simulink model "ekf_simulation"  (R2023a)
settings: Solver=VariableStepAuto  StartTime=0.0  StopTime=3000  RelTol=1e-3  EnableMultiTasking=on
libraries: aausat3_lib x6, simulink_extras x1
settings Model: Creator=brian  LastModifiedBy=jacobel-omar
settings SolverCC: AlgebraicLoopSolver=TrustRegion
settings DataIOCC: SaveFormat=Array  ReturnWorkspaceOutputs=off
settings OptimizationCC: LifeSpan=inf
settings DebuggingCC: SolverPrmCheckMsg=warning  UnconnectedInputMsg=warning  UnconnectedOutputMsg=warning  UnconnectedLineMsg=warning  AllowSymbolicDim=off  SFUnexpectedBacktrackingDiag=warning  SFNoUnconditionalDefaultTransitionDiag=warning  SFExecutionAtInitializationDiag=none  ArithmeticOperatorsInVariantConditions=warning
settings ModelReferenceCC: EnableRefExpFcnMdlSchedulingChecks=on  PropagateSignalLabelsOutOfModel=off
settings SFSimCC: SimUseLocalCustomCode=off  CustomCodeUndefinedFunction=UseInterfaceOnly
settings RTWCC: RTWUseLocalCustomCode=off
settings CodeAppCC: StateflowObjectComments=on
settings GRTTargetCC: TargetLangStandard=C89/C90 (ANSI)
settings ConfigComp: CovMetricSettings=dw  CovSaveCumulativeToWorkspaceVar=on  CovSaveSingleToWorkspaceVar=on  CovExternalEMLEnable=off  CovSFcnEnable=off

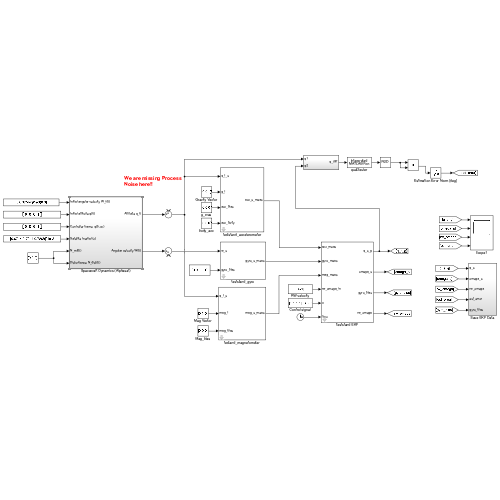
[thumbnail: Simulink's stored preview of the top-level diagram]
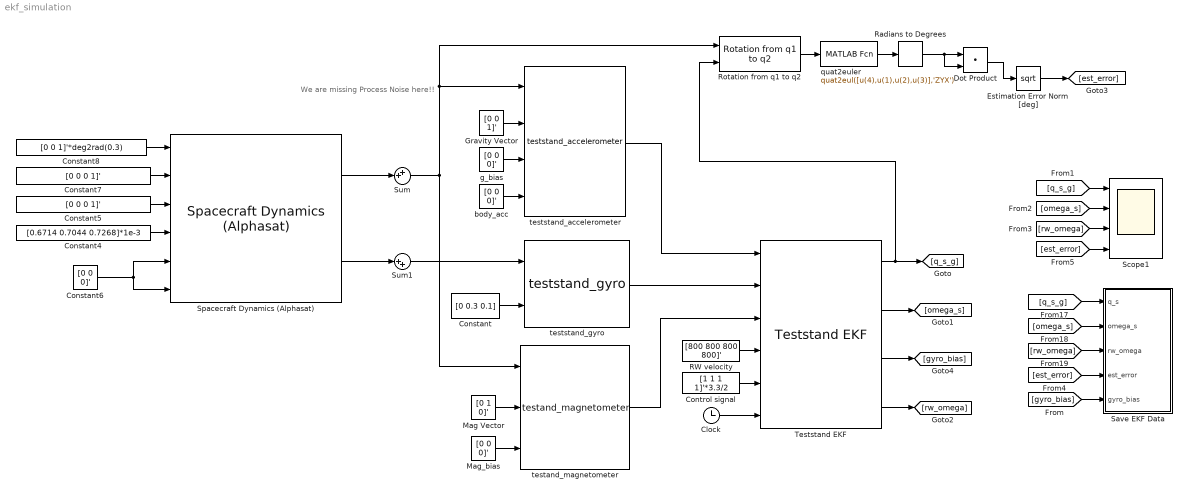
== system ekf_simulation ==
  note: We are missing Process
      | Noise here!!
  Clock : Clock
  Constant : Constant  Value=[0 0.3 0.1]
  Constant4 : Constant  Value=[0.6714 0.7044 0.7268]*1e-3
  Constant5 : Constant  Value=[0 0 0 1]'
  Constant6 : Constant  Value=[0 0 0]'
  Constant7 : Constant  Value=[0 0 0 1]'
  Constant8 : Constant  Value=[0 0 1]'*deg2rad(0.3)
  Control signal : Constant  Value=[1 1 1 1]'*3.3/2
  Dot Product : DotProduct  OutDataTypeStr=Inherit: Inherit via internal rule
  Estimation Error Norm [deg] : Sqrt
  Gravity Vector : Constant  Value=[0 0 1]'  VectorParams1D=off
  Mag Vector : Constant  Value=[0 1 0]'  VectorParams1D=off
  Mag_bias : Constant  Value=[0 0 0]'
  RW velocity : Constant  Value=[800 800 800 800]'
  Radians to Degrees : simulink_extras/Transformations/Radians to Degrees
  Rotation from q1 to q2 : aausat3_lib/Math Utilities/Quaternion operations/Rotation from q1 to q2  SystemSampleTime=-1  VariantActivationTime=update diagram  Latency=0  AutoFrameSizeCalculation=off
      settings: SourceProductName=AAUSAT3
  Save EKF Data : Subsystem
  Scope1 : Scope  NumInputPorts=4
  Spacecraft Dynamics (Alphasat) : aausat3_lib/Dynamics and Kinematics/Spacecraft Dynamics (Alphasat)  SystemSampleTime=-1  VariantActivationTime=update diagram  Latency=0  AutoFrameSizeCalculation=off
      settings: SourceProductName=AAUSAT3
  Sum : Sum  Inputs=++|
  Sum1 : Sum  Inputs=|++
  Teststand EKF : aausat3_lib/ADS/Teststand EKF  dt=0.1  x0=[[0 0 0 1], [0 0 deg2rad(0.03)], [0 0 0], [800 800 800 800]]'  q_s_c=[0 0 0 1]'  q_s_tetra=[0 0 1 0]
      settings: SourceProductName=AAUSAT3
  body_acc : Constant  Value=[0 0 0]'
  g_bias : Constant  Value=[0 0 0]'
  quat2euler : MATLABFcn  MATLABFcn=quat2eul([u(4),u(1),u(2),u(3)],'ZYX')
  testand_magnetometer : aausat3_lib/Sensor Emulation/testand_magnetometer  Ts=-1  mean=0  variance=0.00223  K_factor=eye(3)/0.1465
      settings: SourceProductName=AAUSAT3
  teststand_accelerometer : aausat3_lib/Sensor Emulation/teststand_accelerometer  Ts=-1  mean=0  variance=0.11  K_factor=eye(3)*1/6.1035e-05
      settings: SourceProductName=AAUSAT3
  teststand_gyro : aausat3_lib/Sensor Emulation/teststand_gyro  Ts=-1  mean=0  variance=3.4553109e-6  K_factor=eye(3)/1.3316e-04
      settings: SourceProductName=AAUSAT3
  wires:
  teststand_accelerometer/1 -> Teststand EKF/1
  Mag Vector/1 -> testand_magnetometer/2
  Gravity Vector/1 -> teststand_accelerometer/2
  body_acc/1 -> teststand_accelerometer/4
  Constant4/1 -> Spacecraft Dynamics (Alphasat)/4
  Constant5/1 -> Spacecraft Dynamics (Alphasat)/3
  Constant6/1 -> Spacecraft Dynamics (Alphasat)/6, Spacecraft Dynamics (Alphasat)/5
  Constant7/1 -> Spacecraft Dynamics (Alphasat)/2
  Constant8/1 -> Spacecraft Dynamics (Alphasat)/1
  g_bias/1 -> teststand_accelerometer/3
  Mag_bias/1 -> testand_magnetometer/3
  Teststand EKF/2 -> [omega_s]
  Teststand EKF/1 -> [q_s_g], Rotation from q1 to q2/2
  teststand_gyro/1 -> Teststand EKF/2
  Control signal/1 -> Teststand EKF/5
  Rotation from q1 to q2/1 -> quat2euler/1
  RW velocity/1 -> Teststand EKF/4
  quat2euler/1 -> Radians to Degrees/1
  [q_s_g] -> Save EKF Data/1(q_s)
  [omega_s] -> Save EKF Data/2(omega_s)
  [rw_omega] -> Save EKF Data/3(rw_omega)
  [q_s_g] -> Scope1/1
  [omega_s] -> Scope1/2
  [rw_omega] -> Scope1/3
  [est_error] -> Save EKF Data/4(est_error)
  [est_error] -> Scope1/4
  Sum1/1 -> teststand_gyro/1
  Sum/1 -> testand_magnetometer/1, teststand_accelerometer/1, Rotation from q1 to q2/1
  testand_magnetometer/1 -> Teststand EKF/3
  Clock/1 -> Teststand EKF/6
  Dot Product/1 -> Estimation Error Norm [deg]/1
  Radians to Degrees/1 -> Dot Product/2, Dot Product/1
  Estimation Error Norm [deg]/1 -> [est_error]
  Teststand EKF/4 -> [rw_omega]
  Teststand EKF/3 -> [gyro_bias]
  Constant/1 -> teststand_gyro/2
  Spacecraft Dynamics (Alphasat)/1 -> Sum/2
  Spacecraft Dynamics (Alphasat)/2 -> Sum1/1
  [gyro_bias] -> Save EKF Data/5(gyro_bias)

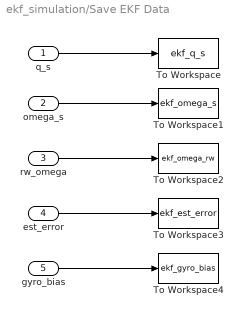
== system ekf_simulation/Save EKF Data ==
  q_s : Inport
  omega_s : Inport  Port=2
  rw_omega : Inport  Port=3
  est_error : Inport  Port=4
  gyro_bias : Inport  Port=5
  To Workspace : ToWorkspace  VariableName=ekf_q_s  SaveFormat=Timeseries  SampleTime=1
  To Workspace1 : ToWorkspace  VariableName=ekf_omega_s  SaveFormat=Timeseries  SampleTime=1
  To Workspace2 : ToWorkspace  VariableName=ekf_omega_rw  SaveFormat=Timeseries  SampleTime=1
  To Workspace3 : ToWorkspace  VariableName=ekf_est_error  SaveFormat=Timeseries  SampleTime=1
  To Workspace4 : ToWorkspace  VariableName=ekf_gyro_bias  SaveFormat=Timeseries  SampleTime=1
  wires:
  q_s/1 -> To Workspace/1
  omega_s/1 -> To Workspace1/1
  rw_omega/1 -> To Workspace2/1
  est_error/1 -> To Workspace3/1
  gyro_bias/1 -> To Workspace4/1
